simulink model "GPCA_Top_Level_Mode_tmp"  (Simulink 8.4)
settings: Solver=ode45  StartTime=0.0  StopTime=10.0  RelTol=1e-3
settings Model: Creator=bourbouh  LastModifiedBy=hbourbou  CovSFcnEnable=on
settings DataIOCC: LimitDataPoints=off  SaveFormat=StructureWithTime  SignalLoggingSaveFormat=Dataset
settings OptimizationCC: ExpressionDepthLimit=128
settings DebuggingCC: UnderspecifiedInitializationDetection=Simplified  MergeDetectMultiDrivingBlocksExec=error  SolverPrmCheckMsg=none  FcnCallInpInsideContextMsg=EnableAllAsError  FrameProcessingCompatibilityMsg=error  StateNameClashWarn=none
settings HardwareCC: ProdBitPerPointer=64  ProdLargestAtomicFloat=Float  ProdIntDivRoundTo=Zero  ProdEndianess=LittleEndian  ProdHWDeviceType=Specified
settings ModelReferenceCC: PropagateSignalLabelsOutOfModel=on
settings GRTTargetCC: CombineOutputUpdateFcns=on  GRTInterface=off

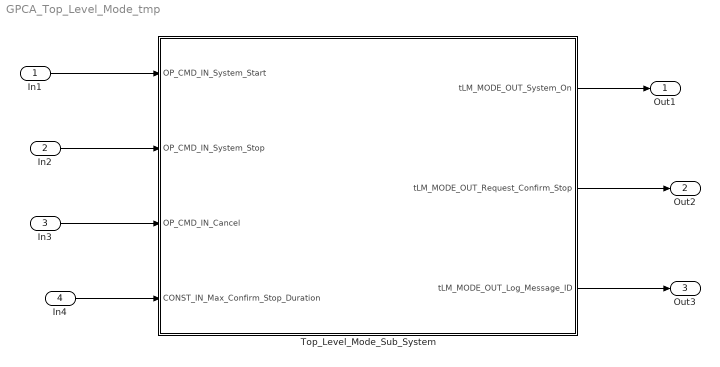
== system GPCA_Top_Level_Mode_tmp ==
  In1 : Inport
  In2 : Inport  Port=2
  In3 : Inport  Port=3
  In4 : Inport  Port=4
  Top_Level_Mode_Sub_System : Stateflow chart  TreatAsAtomicUnit=on
      settings: PermitHierarchicalResolution=ParametersOnly
  Out1 : Outport
  Out2 : Outport  Port=2
  Out3 : Outport  Port=3
  wires:
  In1/1 -> Top_Level_Mode_Sub_System/1(OP_CMD_IN_System_Start)
  In2/1 -> Top_Level_Mode_Sub_System/2(OP_CMD_IN_System_Stop)
  In3/1 -> Top_Level_Mode_Sub_System/3(OP_CMD_IN_Cancel)
  In4/1 -> Top_Level_Mode_Sub_System/4(CONST_IN_Max_Confirm_Stop_Duration)
  Top_Level_Mode_Sub_System/1(tLM_MODE_OUT_System_On) -> Out1/1
  Top_Level_Mode_Sub_System/2(tLM_MODE_OUT_Request_Confirm_Stop) -> Out2/1
  Top_Level_Mode_Sub_System/3(tLM_MODE_OUT_Log_Message_ID) -> Out3/1

== stateflow chart Top_Level_Mode_Sub_System ==
  state TOP_Level_Mode
    entry: tLM_MODE_OUT_System_On=1;
    during: tLM_MODE_OUT_System_On=1;
    exit: tLM_MODE_OUT_System_On=1;
    state Confirm_Stop
      state OFF
        entry:tLM_MODE_OUT_Request_Confirm_Stop=0;
        confirmStopTimer=0;
      state ON
        entry: tLM_MODE_OUT_Request_Confirm_Stop=1;
        confirmStopTimer++;
        during :confirmStopTimer++;
      (default) -> OFF [order 2]
      (default) -> ON [order 1] : [OP_CMD_IN_System_Stop]
      ON -> OFF [order 2] : [OP_CMD_IN_Cancel || confirmStopTimer > Step_Scaling_Factor(CONST_IN_Max_Confirm_Stop_Duration,step_size)]
      OFF -> ON : [OP_CMD_IN_System_Stop]
    (default) -> Confirm_Stop
  state NOT_ON
    entry: tLM_MODE_OUT_System_On=0;
    during: tLM_MODE_OUT_System_On=0;
    exit: tLM_MODE_OUT_System_On=0;
  note: The confirmation to stop the system
      | is abstracted here as !System_Start
  state returnVal = Step_Scaling_Factor(inputVal,step_size) [function]
    (default) -> (junction 20) : {returnVal=inputVal/step_size;}
  state writeLog(logEvent) [function]
    (default) -> (junction 23) : {tLM_MODE_OUT_Log_Message_ID=logEvent;}
  note: step scaling factor returns the scaled time depending upon the step size.
      | If counter has to timeout after 100 seconds and if the step size is 0.1 second
      | the new timeout value = 100/0.1 = 1000 steps.
      | default will be one step = 1 second.
  (default) -> TOP_Level_Mode [order 1] : [OP_CMD_IN_System_Start]
  (default) -> NOT_ON [order 2]
  NOT_ON -> TOP_Level_Mode : [OP_CMD_IN_System_Start]{writeLog(1);}
  ON -> NOT_ON [order 1] : [!OP_CMD_IN_System_Start]{writeLog(2);}
  data: inputVal function_input double; returnVal function_output double; step_size function_input double; logEvent function_input uint8; tLM_MODE_OUT_System_On output boolean; tLM_MODE_OUT_Request_Confirm_Stop output boolean; OP_CMD_IN_System_Start input boolean; OP_CMD_IN_System_Stop input boolean; OP_CMD_IN_Cancel input boolean; CONST_IN_Max_Confirm_Stop_Duration input double; step_size parameter double; tLM_MODE_OUT_Log_Message_ID output uint8; confirmStopTimer local double
